simulink model "velocity_profile"  (R2019b)
settings: Solver=FixedStepAuto  StartTime=0.0  StopTime=500  FixedStep=0.1  RelTol=1e-3
libraries: simulink x1
settings Model: Creator=LimingGao  LastModifiedBy=LimingGao
settings DataIOCC: ReturnWorkspaceOutputs=off

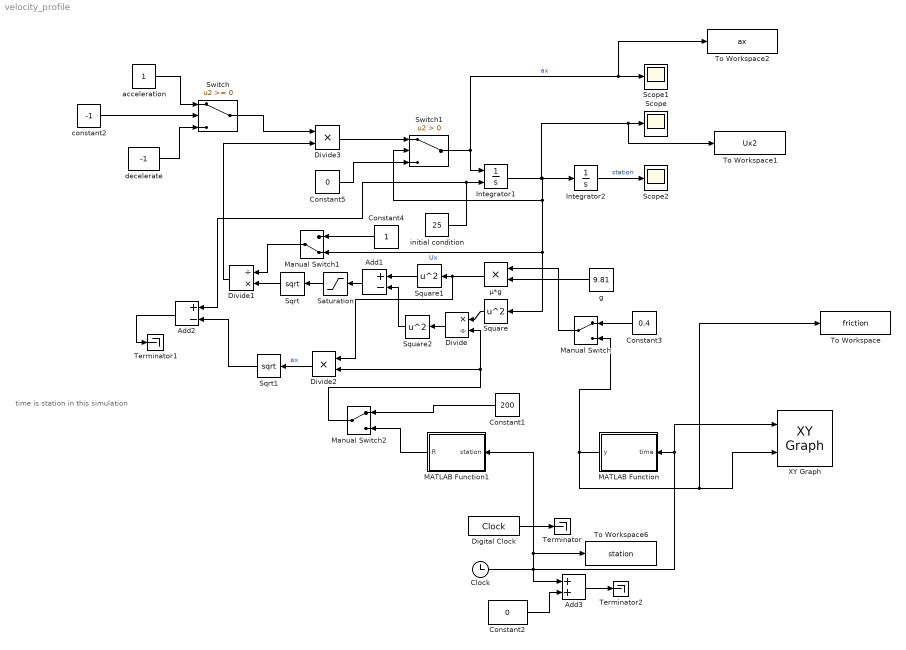
== system velocity_profile ==
  note: time is station in this simulation
  Add1 : Sum  Inputs=+-
  Add2 : Sum  Inputs=+-
  Add3 : Sum
  Clock : Clock
  Constant1 : Constant  Value=200
  Constant2 : Constant  Value=0
  Constant3 : Constant  Value=0.4
  Constant4 : Constant
  Constant5 : Constant  Value=0
  Digital Clock : DigitalClock  SampleTime=0.1
  Divide : Product  Inputs=*/
  Divide1 : Product  Inputs=/*
  Divide2 : Product  Inputs=**
  Divide3 : Product  Inputs=**
  Integrator1 : Integrator  InitialConditionSource=external  InitialCondition=20
  Integrator2 : Integrator
  MATLAB Function : MATLAB Function  TreatAsAtomicUnit=on
      settings: AttributesFormatString=%<SystemSampleTime>
  MATLAB Function1 : MATLAB Function  TreatAsAtomicUnit=on
      settings: AttributesFormatString=%<SystemSampleTime>
  Manual Switch : ManualSwitch
  Manual Switch1 : ManualSwitch  CurrentSetting=0
  Manual Switch2 : ManualSwitch
  Saturation : Saturate  UpperLimit=+inf  LowerLimit=0
  Scope : Scope
  Scope1 : Scope
  Scope2 : Scope
  Sqrt : Sqrt  SaturateOnIntegerOverflow=on
  Sqrt1 : Sqrt  SaturateOnIntegerOverflow=on
  Square : Math  Operator=square  SignedPower=off  SaturateOnIntegerOverflow=on
  Square1 : Math  Operator=square  SignedPower=off  SaturateOnIntegerOverflow=on
  Square2 : Math  Operator=square  SignedPower=off  SaturateOnIntegerOverflow=on
  Switch : Switch
  Switch1 : Switch  Criteria=u2 > Threshold
  Terminator : Terminator
  Terminator1 : Terminator
  Terminator2 : Terminator
  To Workspace : ToWorkspace  VariableName=friction  SampleTime=-1
  To Workspace1 : ToWorkspace  VariableName=Ux2  SampleTime=-1
  To Workspace2 : ToWorkspace  VariableName=ax  SampleTime=-1
  To Workspace6 : ToWorkspace  VariableName=station  SampleTime=-1
      settings: Save2DSignal=2-D array (concatenate along first dimension)
  XY Graph : simulink/Sinks/XY Graph  xmin=-1  xmax=500  ymin=0  ymax=1  st=-1
  acceleration : Constant
  constant2 : Constant  Value=-1
  decelerate : Constant  Value=-1
  g : Constant  Value=9.81
  initial condition : Constant  Value=25
  μ*g : Product  Inputs=**
  wires:
  Divide1/1 -> Divide3/2
  Integrator1/1 -> Integrator2/1, Manual Switch1/2, Square/1, Switch1/2, To Workspace1/1, Scope/1  "Ux"
  Square1/1 -> Add1/1
  μ*g/1 -> Divide2/1, Square1/1
  Add1/1 -> Saturation/1
  Square/1 -> Divide/1
  Manual Switch2/1 -> Divide2/2, Divide/2
  Divide/1 -> Square2/1
  Square2/1 -> Add1/2
  Sqrt/1 -> Divide1/2
  Saturation/1 -> Sqrt/1
  initial condition/1 -> Add2/1, Integrator1/2
  Divide2/1 -> Sqrt1/1  "ax"
  Sqrt1/1 -> Add2/2
  acceleration/1 -> Switch/1
  Switch/1 -> Divide3/1
  decelerate/1 -> Switch/3
  g/1 -> μ*g/2
  Clock/1 -> MATLAB Function1/1(station), To Workspace6/1, Add3/1, XY Graph/1, MATLAB Function/1(time)
  Constant2/1 -> Add3/2
  Digital Clock/1 -> Terminator/1
  Constant3/1 -> Manual Switch/1
  Manual Switch/1 -> μ*g/1
  MATLAB Function/1(y) -> To Workspace/1, XY Graph/2, Manual Switch/2
  constant2/1 -> Switch/2
  Add2/1 -> Terminator1/1
  Divide3/1 -> Switch1/1
  Switch1/1 -> Integrator1/1, To Workspace2/1, Scope1/1  "ax"
  Constant5/1 -> Switch1/3
  Integrator2/1 -> Scope2/1  "station"
  Add3/1 -> Terminator2/1
  Constant4/1 -> Manual Switch1/1
  Manual Switch1/1 -> Divide1/1
  MATLAB Function1/1(R) -> Manual Switch2/2
  Constant1/1 -> Manual Switch2/1

== matlab function velocity_profile/MATLAB Function1 ==
  data: R output; station input
% Purpose: calculate some friction data
% input: time
%
% ouput: friction data of 4 wheels

function R = radius_generator(station)

% Initialization
%A persistent variable is a local variable in a MATLAB function that retains
% its value in memory between calls to the function.
% For code generation, functions must initialize a persistent variable if it is empty.
R = 200-2.5*station;
    
end

== matlab function velocity_profile/MATLAB Function ==
  data: y output; time input
% Purpose: calculate some friction data
% input: time
%
% ouput: friction data of 4 wheels

function y = fric_generator(time)

% Initialization
%A persistent variable is a local variable in a MATLAB function that retains
% its value in memory between calls to the function.
% For code generation, functions must initialize a persistent variable if it is empty.
if time< 200
    y = 0.9;
elseif time>= 200 && time< 300
    y = 0.4;
elseif time>= 300 && time< 500
    y = 0.9;
else
    y = (0.85+0.15*sin(time*2*pi/200));
    
end
